simulink model "Multiplier16x16"  (R2022b)
settings: Solver=VariableStepAuto  StartTime=0.0  StopTime=10.0  RelTol=1e-3
libraries: raspberrypiIOTlib x4, raspberrypiCommlib x3, simulink x1
settings Model: Creator=pezz9  LastModifiedBy=pezz9

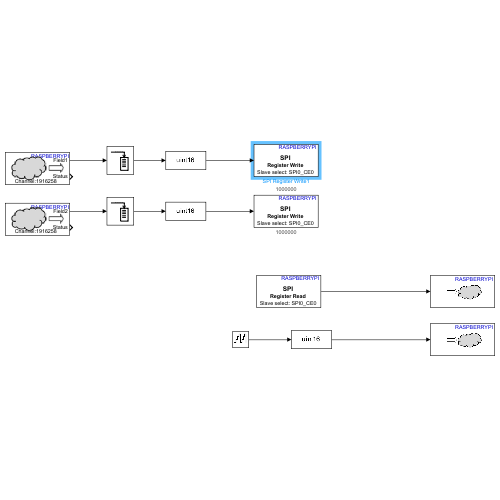
[thumbnail: Simulink's stored preview of the top-level diagram]
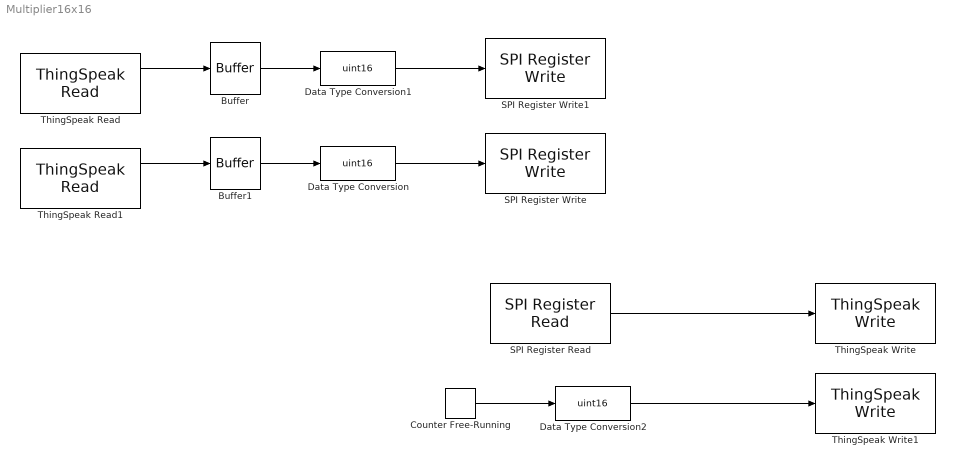
== system Multiplier16x16 ==
  Buffer : Buffer  N=128  OutputFrames=off
  Buffer1 : Buffer  N=128  OutputFrames=off
  Counter Free-Running : simulink/Sources/Counter Free-Running  NumBits=16  tsamp=-1
  Data Type Conversion : DataTypeConversion  OutDataTypeStr=uint16  RndMeth=Floor
  Data Type Conversion1 : DataTypeConversion  OutDataTypeStr=uint16  RndMeth=Floor
  Data Type Conversion2 : DataTypeConversion  OutDataTypeStr=uint16  RndMeth=Floor
  SPI Register Read : raspberrypiCommlib/SPI Register Read  BoardProperty=Pi 2 Model B  SSPin=SPI0_CE0  SPIModule=uint32(0)  Mode=Master  BusSpeed=1000000  Pin=uint32(0)  FirstBitToTransfer=Most significant bit (MSB)  ClockMode=1  BlockFunction=Read  RegisterAddress=0  OutputDataType=uint32  OutputDataLength=1  SampleTime=0.1
  SPI Register Write : raspberrypiCommlib/SPI Register Write  BoardProperty=Pi 2 Model B  SSPin=SPI0_CE0  SPIModule=uint32(0)  Mode=Master  BusSpeed=1000000  Pin=uint32(0)  FirstBitToTransfer=Most significant bit (MSB)  ClockMode=1  BlockFunction=Write  RegisterAddress=0  OutputDataType=int8  OutputDataLength=1
      settings: AttributesFormatString=%<BusSpeed>
  SPI Register Write1 : raspberrypiCommlib/SPI Register Write  BoardProperty=Pi 2 Model B  SSPin=SPI0_CE0  SPIModule=uint32(0)  Mode=Master  BusSpeed=1000000  Pin=uint32(0)  FirstBitToTransfer=Most significant bit (MSB)  ClockMode=1  BlockFunction=Write  RegisterAddress=0  OutputDataType=int8  OutputDataLength=1
      settings: AttributesFormatString=%<BusSpeed>
  ThingSpeak Read : raspberrypiIOTlib/ThingSpeak Read  ChannelID=1916258  ChannelAccess=Private  ReadAPIKey=D0EVAQ5KG83O8BJ8  FieldNumber=1  PrintDiagnosticMessages=off  SampleTime=60  blockPlatform=LINUX
  ThingSpeak Read1 : raspberrypiIOTlib/ThingSpeak Read  ChannelID=1916258  ChannelAccess=Private  ReadAPIKey=D0EVAQ5KG83O8BJ8  FieldNumber=2  PrintDiagnosticMessages=off  SampleTime=60  blockPlatform=LINUX
  ThingSpeak Write : raspberrypiIOTlib/ThingSpeak Write  UpdateURL=https://api.thingspeak.com/update  WriteAPIKey=ISCNEIZY65FPF4J2  NumberOfFields=1  UpdateInterval=60  PrintDiagnosticMessages=off  CoordinatesEnabled=off  CoordSrc=Block dialog  Coordinates=[42.29971, -71.350719, 69.29]  blockPlatform=Raspberry Pi
  ThingSpeak Write1 : raspberrypiIOTlib/ThingSpeak Write  UpdateURL=https://api.thingspeak.com/update  WriteAPIKey=ISCNEIZY65FPF4J2  NumberOfFields=1  UpdateInterval=60  PrintDiagnosticMessages=off  CoordinatesEnabled=off  CoordSrc=Block dialog  Coordinates=[42.29971, -71.350719, 69.29]  blockPlatform=Raspberry Pi
  wires:
  Buffer/1 -> Data Type Conversion1/1
  Buffer1/1 -> Data Type Conversion/1
  ThingSpeak Read1/1 -> Buffer1/1
  ThingSpeak Read/1 -> Buffer/1
  Data Type Conversion/1 -> SPI Register Write/1
  Data Type Conversion1/1 -> SPI Register Write1/1
  SPI Register Read/1 -> ThingSpeak Write/1
  Data Type Conversion2/1 -> ThingSpeak Write1/1
  Counter Free-Running/1 -> Data Type Conversion2/1
